simulink model "Lidar_System_July03_v1"  (Simulink 7.3)
settings: Solver=FixedStepDiscrete  StartTime=0.0  StopTime=inf  FixedStep=0.1  MaxStep=0.2  RelTol=1e-3
undefined symbols (not defined in the file): strel
libraries: dspmtrx3 x86, simulink x64, dspstat3 x37, vipstatistics x15, vipmorphops x15
(part 8 of 8)

== matlab function Enabled Subsystem1/Perception/Color Analysis/Template Matching (Docking)/Blue/Triangle/Docking1/Recognition/Embedded MATLAB Function ==
  data: targetTemp input double; bbox_out output double; cruciform input double; circle input double; triangle input double; whitePixCount input double; threshold input double; V_mask input double; bbox_in input double; returnRatioDiff output double
function [bbox_out,returnRatioDiff] = recognition(targetTemp,cruciform,circle,triangle,...
    whitePixCount,threshold,V_mask,bbox_in)

% Written by Edward Zhu on 5/14/14

% Inputs
% tempID:       Number corresponding to one of the templates (cruciform: 1,
%               circle: 2, triangle: 3)
% cruciform:    19*19 template of cruciform
% circle:       19*19 template of circle
% triangle:     19*19 template of triangle
% whitePixCount:Number of white pixels in each of the templates
% V_mask:       V channel binary mask
% bbox_in:      Bounding boxes as found by blob analysis
% label:        Label matrix as found by blob analysis

% Outputs
% bbox_out:     Bounding box of matched symbol
% symFound:     Status of matching (found: 1, not found: 0)

% Define frame and template size
templates = zeros(19,19,3);
templates(:,:,1) = cruciform;
templates(:,:,2) = circle;
templates(:,:,3) = triangle;
templates = 2*(templates-0.5);

tempRows = size(templates,1);
tempCols = size(templates,2);
numBBox = size(bbox_in,1);

% Initialize scaled image and output bbox matrices
V_scaled = zeros(tempRows,tempCols);
bbox_out = uint32(zeros(numBBox,4));

returnRatioDiff = ones(numBBox,1);

for i = 1:numBBox
       
    if (min(bbox_in(i,:)) > 0 && (bbox_in(i,1)+bbox_in(i,3)) < 640  && (bbox_in(i,2) + bbox_in(i,4) < 480))
        similarity = 0;
        rowScaleStep = floor(bbox_in(i,4) / tempRows);
        colScaleStep = floor(bbox_in(i,3) / tempCols);
        
        captureRow = bbox_in(i,2);
        for row = 1:tempRows
            captureCol = bbox_in(i,1);
            if (captureCol > 640)
                captureCol = uint32(640);
            end
            if (captureRow > 480)
                captureRow = uint32(480);
            end
            for col = 1:tempCols
                V_scaled(row,col) = V_mask(captureRow,captureCol);
                similarity = similarity + templates(row,col,targetTemp) * (V_mask(captureRow,captureCol)*(-1) + 1);
                captureCol = captureCol + colScaleStep;
            end
            captureRow = captureRow + rowScaleStep;
        end
        
        ratioDiff = abs(1 - single(similarity) / single(whitePixCount(targetTemp)));
        
        % Output valid bounding box
        if ratioDiff < threshold
            bbox_out(i,:) = bbox_in(i,:);
            returnRatioDiff(i) = ratioDiff;
        end
    end
end

== matlab function Enabled Subsystem1/Perception/Color Analysis/Template Matching (Docking)/Black/Embedded MATLAB Function ==
  data: mode input double; CrucEn output double; CircleEn output double; TriEn output double
function [CrucEn,CircleEn,TriEn] = ShapeEnabler(mode)

CrucEn=0;
CircleEn=0;
TriEn=0;

if mode ==14 ;
    CrucEn=1;
elseif mode == 15;
    CircleEn=1;
else
    TriEn=1;
end

end

== matlab function Enabled Subsystem1/Perception/Color Analysis/Template Matching (Docking)/Black/Triangle/Docking1/BBox Transform ==
  data: BBin input double; BBout output double
function BBout = Btrans(BBin)
%Change BBbox from 2009 layout to 2014 layout to work with other code

BBinT = BBin';

r1 = BBinT(2,:);
c1 = BBinT(1,:);
h1 = BBinT(4,:);
w1 = BBinT(3,:);

% x1 = BBinT(:,2);
% y1 = BBinT(:,1);
% h1 = BBinT(:,3);
% w1 = BBinT(:,4);

BBout = [r1;c1;h1;w1];
%BBout = [x1 y1 w1 h1];

== matlab function Enabled Subsystem1/Perception/Color Analysis/Template Matching (Docking)/Black/Triangle/Docking1/Blob Analysis/BBox Transform ==
  data: BBin input double; BBout output double
function BBout = Btrans(BBin)
%Change BBbox from 2009 layout to 2014 layout to work with other code

BBinT = BBin';

x1 = BBinT(:,2);
y1 = BBinT(:,1);
h1 = BBinT(:,3);
w1 = BBinT(:,4);

BBout = [x1 y1 w1 h1];

== matlab function Enabled Subsystem1/Perception/Color Analysis/Template Matching (Docking)/Black/Triangle/Docking1/Detection/Detection ==
  data: cruciform input double; bbox_out output double; circle input double; triangle input double; whitePixCount input double; threshold input double; V_mask input double; bbox_in input double; label input double; rtnRatioDiff output double
function [bbox_out,rtnRatioDiff]= detection(cruciform,circle,triangle,...
    whitePixCount,threshold,V_mask,bbox_in,label)

% Written by Edward Zhu on 5/14/14

% Inputs
% tempID:       Number corresponding to one of the templates (cruciform: 1,
%               circle: 2, triangle: 3)
% cruciform:    19*19 template of cruciform
% circle:       19*19 template of circle
% triangle:     19*19 template of triangle
% whitePixCount:Number of white pixels in each of the templates
% V_mask:       V channel binary mask
% bbox_in:      Bounding boxes as found by blob analysis
% label:        Label matrix as found by blob analysis

% Outputs
% bbox_out:     Bounding box of matched symbol
% symFound:     Status of matching (found: 1, not found: 0)

% Define frame and template size
templates = zeros(19,19,3);
templates(:,:,1) = cruciform;
templates(:,:,2) = circle;
templates(:,:,3) = triangle;

imgRows = size(label,1);
imgCols = size(label,2);
tempRows = size(templates,1);
tempCols = size(templates,2);
numBBox = size(bbox_in,1);

% Initialize scaled image and output bbox matrices
V_scaled = zeros(tempRows,tempCols);
bbox_out = uint32(zeros(numBBox,4));
rtnRatioDiff = ones(numBBox,1);

bestRatioDiff = single(1);

for i = 1:numBBox
    shapeDiff = abs(1-bbox_in(i,3)/bbox_in(i,4));
    if bbox_in(i,3) >= tempCols && bbox_in(i,4) >= tempRows && shapeDiff < 0.5
        % Set up arrays for the start and end rows and columns for bbox
        % matching
        
        similarity = zeros(1,3);
        ratioDiff = zeros(1,3);
        
        rowStep = floor(bbox_in(i,4) / tempRows);
        colStep = floor(bbox_in(i,3) / tempCols);
        
        startRowList = zeros(1,3);
        startRowList(2) = bbox_in(i,2);
        startRowList(1) = max(1, startRowList(2) - rowStep);
        startRowList(3) = min(imgRows, startRowList(2) + rowStep);
        
        endRowList = zeros(1,3);
        endRowList(2) = bbox_in(i,2) + bbox_in(i,4);
        endRowList(1) = max(1, endRowList(2) - rowStep);
        endRowList(3) = min(imgRows, endRowList(2) + rowStep);
        
        startColList = zeros(1,3);
        startColList(2) = bbox_in(i,1);
        startColList(1) = max(1, startColList(2) - colStep);
        startColList(3) = min(imgCols, startColList(2) + colStep);
        
        endColList = zeros(1,3);
        endColList(2) = bbox_in(i,1) + bbox_in(i,3);
        endColList(1) = max(1, endColList(2) - colStep);
        endColList(3) = min(imgCols, endColList(2) + colStep);
        
        % Scale down image in bbox to size of template (18*18 px)
        for startRow = startRowList
            for endRow = endRowList
                rowScaleStep = floor((endRow - startRow) / tempRows);
                
                for startCol = startColList
                    for endCol = endColList
                        colScaleStep = floor((endCol - startCol) / tempCols);
                        
                        captureRow = startRow;
                        for row = 1:tempRows
                            captureCol = startCol;
                            for col = 1:tempCols
                                V_scaled(row,col) = V_mask(captureRow,captureCol);
                                for tempID = 1:3
                                    similarity(tempID) = similarity(tempID) + templates(row,col,tempID) * (V_mask(captureRow,captureCol)*(-1) + 1);
                                end
                                captureCol = captureCol + colScaleStep;                        
                            end
                            captureRow = captureRow + rowScaleStep;
                        end                  
                        
                        for tempID = 1:3   
                            ratioDiff(tempID) = abs(1 - single(similarity(tempID)) / single(whitePixCount(tempID))); 
                        end
                        
                        if min(ratioDiff) < bestRatioDiff
                            bestRatioDiff = single(min(ratioDiff));
                        end
                    end
                end
            end
        end
        
        % Output valid bounding boxes
        if bestRatioDiff < threshold
            bbox_out(i,:) = bbox_in(i,:);
            rtnRatioDiff(i) = bestRatioDiff;
        end
    end
end

== matlab function Enabled Subsystem1/Perception/Color Analysis/Template Matching (Docking)/Black/Triangle/Docking1/Embedded MATLAB Function ==
  data: xRec input double; bayNumber output double; xDet input double
function bayNumber = bayPosition(xRec,xDet)

symxpos = xRec(1);

diff1 = xDet(1) - symxpos;
diff2 = xDet(2) - symxpos;
diff3 = xDet(3) - symxpos;

if diff1 == 0
    bayNumber = uint8(1);
elseif diff2 == 0
    bayNumber = uint8(2);
elseif diff3 == 0
    bayNumber = uint8(3);
else
    bayNumber = uint8(0);
end

== matlab function Enabled Subsystem1/Perception/Color Analysis/Template Matching (Docking)/Black/Triangle/Docking1/Embedded MATLAB Function1 ==
  data: uv_d input double; Distances output double; BBox input double; Angles output double
function [Distances, Angles]  = DsitFind(uv_d,BBox)

% Based on the location of the signs find their distance

% Predefine output distance matrix
Distances = zeros(4,1);
Angles = zeros(4,1);

% Parse BBox information
xpos = BBox(1,1);
ypos = BBox(1,2);
width = BBox(1,3);
height = BBox(1,4);

% Zero count and total of distance measurements
count = 0;
total = 0;

for i = ypos:(ypos+height)
    for j = xpos:(xpos+width)
        % Find total number of points in box where distance value has
        % been gathered and total of all distance in box
        if (uv_d(i,j) > 1)
            count = count+1;
            total = total+uv_d(i,j);
        end
    end
end

% Find average value of nonzero elements inside BBox
Distances(1,1) = round(total/(count*10));
Angles(1,1) = ((xpos + width)/2-3.135858904821101e+02)/554.8582*180/pi;


end

== matlab function Enabled Subsystem1/Perception/Color Analysis/Template Matching (Docking)/Black/Triangle/Docking1/Recognition/Embedded MATLAB Function ==
  data: targetTemp input double; bbox_out output double; cruciform input double; circle input double; triangle input double; whitePixCount input double; threshold input double; V_mask input double; bbox_in input double; returnRatioDiff output double
function [bbox_out,returnRatioDiff] = recognition(targetTemp,cruciform,circle,triangle,...
    whitePixCount,threshold,V_mask,bbox_in)

% Written by Edward Zhu on 5/14/14

% Inputs
% tempID:       Number corresponding to one of the templates (cruciform: 1,
%               circle: 2, triangle: 3)
% cruciform:    19*19 template of cruciform
% circle:       19*19 template of circle
% triangle:     19*19 template of triangle
% whitePixCount:Number of white pixels in each of the templates
% V_mask:       V channel binary mask
% bbox_in:      Bounding boxes as found by blob analysis
% label:        Label matrix as found by blob analysis

% Outputs
% bbox_out:     Bounding box of matched symbol
% symFound:     Status of matching (found: 1, not found: 0)

% Define frame and template size
templates = zeros(19,19,3);
templates(:,:,1) = cruciform;
templates(:,:,2) = circle;
templates(:,:,3) = triangle;
templates = 2*(templates-0.5);

tempRows = size(templates,1);
tempCols = size(templates,2);
numBBox = size(bbox_in,1);

% Initialize scaled image and output bbox matrices
V_scaled = zeros(tempRows,tempCols);
bbox_out = uint32(zeros(numBBox,4));

returnRatioDiff = ones(numBBox,1);

for i = 1:numBBox
       
    if (min(bbox_in(i,:)) > 0 && (bbox_in(i,1)+bbox_in(i,3)) < 640  && (bbox_in(i,2) + bbox_in(i,4) < 480))
        similarity = 0;
        rowScaleStep = floor(bbox_in(i,4) / tempRows);
        colScaleStep = floor(bbox_in(i,3) / tempCols);
        
        captureRow = bbox_in(i,2);
        for row = 1:tempRows
            captureCol = bbox_in(i,1);
            if (captureCol > 640)
                captureCol = uint32(640);
            end
            if (captureRow > 480)
                captureRow = uint32(480);
            end
            for col = 1:tempCols
                V_scaled(row,col) = V_mask(captureRow,captureCol);
                similarity = similarity + templates(row,col,targetTemp) * (V_mask(captureRow,captureCol)*(-1) + 1);
                captureCol = captureCol + colScaleStep;
            end
            captureRow = captureRow + rowScaleStep;
        end
        
        ratioDiff = abs(1 - single(similarity) / single(whitePixCount(targetTemp)));
        
        % Output valid bounding box
        if ratioDiff < threshold
            bbox_out(i,:) = bbox_in(i,:);
            returnRatioDiff(i) = ratioDiff;
        end
    end
end
